simulink model "DEF_IEEE14_case3"  (R2023b)
settings: Solver=FixedStepAuto  StartTime=0  StopTime=30  FixedStep=Ts  RelTol=1e-3
StopFcn:
  | %data_idq_all = out.data_idq_all;
  | %save('Oscillation_July\data\data_idq_all.mat','data_idq_all');
  | %data_vdq_all = out.data_vdq_all;
  | %save('Oscillation_July\data\data_vdq_all.mat','data_vdq_all');
values from neighbouring files (symbols this model uses):
  freq_sel = imag(Mode_Hz)    [Mode_Right_Eig.m]
  Mode_Rad = D(ModeSel, ModeSel)    [Mode_Right_Eig.m]
undefined symbols (not defined in the file or in its folder): ApparatusDiscreDamping, ApparatusPara, ApparatusPowerFlow, ApparatusType, DiscIntNeverNeededParam, Fbase, fpll, k_lpf, lpf_A, lpf_B, lpf_C, lpf_D, OtherInputs, Sbase, Tdef_start, Ts, Vbase, Wbase, wc_lpf, x_e, Ybase, Zbase
libraries: SimplusGT x46, spsGroundLib x22, spsThreePhaseSeriesRLCBranchLib x20, spsThreePhaseParallelRLCBranchLib x14, spsThreePhaseTransformerTwoWindingsLib x3, eeGeneralControl x2, spsFourierLib x2, spspowerguiLib x1
(part 3 of 3)

== system DEF_IEEE14_case3/uDEF8/PI ==
  e : Inport
  Discrete-Time Integrator : DiscreteIntegrator  gainval=1  InitialCondition=2*pi*Fbase  SampleTime=Ts  LimitOutput=on  UpperSaturationLimit=2*pi*Fbase + IntSat_PLL  LowerSaturationLimit=2*pi*Fbase - IntSat_PLL  ICPrevOutput=DiscIntNeverNeededParam  ICPrevScaledInput=DiscIntNeverNeededParam
  Ki : Gain  Gain=Ki_PLL  SaturateOnIntegerOverflow=on  OutDataTypeStr=Inherit: Same as input  ParamDataTypeStr=Inherit: Same as input
  Kp : Gain  Gain=Kp_PLL  SaturateOnIntegerOverflow=on  OutDataTypeStr=Inherit: Same as input  ParamDataTypeStr=Inherit: Same as input
  Sum4 : Sum  SaturateOnIntegerOverflow=on
  Out : Outport
  wires:
  Sum4/1 -> Out/1
  Discrete-Time Integrator/1 -> Sum4/2
  e/1 -> Kp/1, Ki/1
  Kp/1 -> Sum4/1
  Ki/1 -> Discrete-Time Integrator/1

== system DEF_IEEE14_case3/uDEF9/Initial_filter4 ==
  original : Inport
  Clock1 : Clock
  Gain7 : Gain
  Gain8 : Gain  Gain=0
  Switch3 : Switch  Criteria=u2 > Threshold  Threshold=Tdef_start  SaturateOnIntegerOverflow=off  InputSameDT=off
  filtered : Outport
  wires:
  Switch3/1 -> filtered/1  "dTheta"
  original/1 -> Gain8/1, Gain7/1
  Gain7/1 -> Switch3/1
  Gain8/1 -> Switch3/3
  Clock1/1 -> Switch3/2

== system DEF_IEEE14_case3/uDEF9/Initial_filter5 ==
  original : Inport
  Clock1 : Clock
  Gain7 : Gain
  Gain8 : Gain  Gain=0
  Switch3 : Switch  Criteria=u2 > Threshold  Threshold=Tdef_start  SaturateOnIntegerOverflow=off  InputSameDT=off
  filtered : Outport
  wires:
  Switch3/1 -> filtered/1  "dTheta"
  original/1 -> Gain8/1, Gain7/1
  Gain7/1 -> Switch3/1
  Gain8/1 -> Switch3/3
  Clock1/1 -> Switch3/2

== system DEF_IEEE14_case3/uDEF9/Initial_filter6 ==
  original : Inport
  Clock1 : Clock
  Gain7 : Gain
  Gain8 : Gain  Gain=0
  Switch3 : Switch  Criteria=u2 > Threshold  Threshold=Tdef_start  SaturateOnIntegerOverflow=off  InputSameDT=off
  filtered : Outport
  wires:
  Switch3/1 -> filtered/1  "dTheta"
  original/1 -> Gain8/1, Gain7/1
  Gain7/1 -> Switch3/1
  Gain8/1 -> Switch3/3
  Clock1/1 -> Switch3/2

== system DEF_IEEE14_case3/uDEF9/Initial_filter7 ==
  original : Inport
  Clock1 : Clock
  Gain7 : Gain
  Gain8 : Gain  Gain=0
  Switch3 : Switch  Criteria=u2 > Threshold  Threshold=Tdef_start  SaturateOnIntegerOverflow=off  InputSameDT=off
  filtered : Outport
  wires:
  Switch3/1 -> filtered/1  "dTheta"
  original/1 -> Gain8/1, Gain7/1
  Gain7/1 -> Switch3/1
  Gain8/1 -> Switch3/3
  Clock1/1 -> Switch3/2

== system DEF_IEEE14_case3/uDEF9/Initial_filter8 ==
  original : Inport
  Clock1 : Clock
  Gain7 : Gain
  Gain8 : Gain  Gain=0
  Switch3 : Switch  Criteria=u2 > Threshold  Threshold=Tdef_start  SaturateOnIntegerOverflow=off  InputSameDT=off
  filtered : Outport
  wires:
  Switch3/1 -> filtered/1  "dTheta"
  original/1 -> Gain8/1, Gain7/1
  Gain7/1 -> Switch3/1
  Gain8/1 -> Switch3/3
  Clock1/1 -> Switch3/2

== system DEF_IEEE14_case3/uDEF9/Initial_filter9 ==
  original : Inport
  Clock1 : Clock
  Gain7 : Gain
  Gain8 : Gain  Gain=0
  Switch3 : Switch  Criteria=u2 > Threshold  Threshold=Tdef_start  SaturateOnIntegerOverflow=off  InputSameDT=off
  filtered : Outport
  wires:
  Switch3/1 -> filtered/1  "dTheta"
  original/1 -> Gain8/1, Gain7/1
  Gain7/1 -> Switch3/1
  Gain8/1 -> Switch3/3
  Clock1/1 -> Switch3/2

== system DEF_IEEE14_case3/uDEF9/PI ==
  e : Inport
  Discrete-Time Integrator : DiscreteIntegrator  gainval=1  InitialCondition=2*pi*Fbase  SampleTime=Ts  LimitOutput=on  UpperSaturationLimit=2*pi*Fbase + IntSat_PLL  LowerSaturationLimit=2*pi*Fbase - IntSat_PLL  ICPrevOutput=DiscIntNeverNeededParam  ICPrevScaledInput=DiscIntNeverNeededParam
  Ki : Gain  Gain=Ki_PLL  SaturateOnIntegerOverflow=on  OutDataTypeStr=Inherit: Same as input  ParamDataTypeStr=Inherit: Same as input
  Kp : Gain  Gain=Kp_PLL  SaturateOnIntegerOverflow=on  OutDataTypeStr=Inherit: Same as input  ParamDataTypeStr=Inherit: Same as input
  Sum4 : Sum  SaturateOnIntegerOverflow=on
  Out : Outport
  wires:
  Ki/1 -> Discrete-Time Integrator/1
  Kp/1 -> Sum4/1
  e/1 -> Ki/1, Kp/1
  Discrete-Time Integrator/1 -> Sum4/2
  Sum4/1 -> Out/1
